simulink model "w3_warplab_trigger_proc"  (Simulink 7.7)
settings: Solver=ode45  StartTime=0.0  StopTime=100  RelTol=1e-3
InitFcn:
  | warplab_trigger_proc_init
StartFcn:
  | warplab_trigger_proc_init
undefined symbols (not defined in the file or in its folder): gcbh, xlBlockLoadCallback, xlGetNormalizedPeriod
libraries: xbsIndex_r4 x817, xbsEDKLib_r4 x1
(part 6 of 6)

== system w3_warplab_trigger_proc/Trigger Sources/Energy/AntD Detector/Idle Detection ==
  Avg RSSI : Inport
  Reset : Inport  Port=2
  en : Inport  Port=3
  Convert1 : xbsIndex_r4/Convert  gui_display_data_type=Fixed-point  arith_type=Unsigned  n_bits=1  bin_pt=0  float_type=Single  exp_bits=8  fraction_bits=24  quantization=Truncate  overflow=Wrap  en=off  latency=0  dbl_ovrd=off  pipeline=off  block_type=convert
      settings: block_version=VER_STRING_GOES_HERE
  Counter1 : xbsIndex_r4/Counter  cnt_type=Free Running  cnt_to=Inf  operation=Up  start_count=0  cnt_by_val=1  arith_type=Unsigned  n_bits=11  bin_pt=0  load_pin=off  rst=on  en=on  explicit_period=off  period=4  dbl_ovrd=off  use_behavioral_HDL=off  implementation=Fabric  use_rpm=off  block_type=counter
  Inverter1 : xbsIndex_r4/Inverter  en=off  latency=0  dbl_ovrd=off  block_type=inv
      settings: xl_area=[0 0 0 0 0 0 0]  block_version=8.2
  Logical : xbsIndex_r4/Logical  logical_function=AND  inputs=2  en=off  latency=0  precision=Full  arith_type=Unsigned  n_bits=16  bin_pt=0  align_bp=on  dbl_ovrd=off  block_type=logical
  Logical1 : xbsIndex_r4/Logical  logical_function=OR  inputs=2  en=off  latency=0  precision=Full  arith_type=Unsigned  n_bits=16  bin_pt=0  align_bp=on  dbl_ovrd=off  block_type=logical
  Relational2 : xbsIndex_r4/Relational  mode=a<b  en=off  latency=0  dbl_ovrd=off  block_type=relational
      settings: block_version=VER_STRING_GOES_HERE
  Relational3 : xbsIndex_r4/Relational  mode=a>b  en=off  latency=0  dbl_ovrd=off  block_type=relational
      settings: block_version=VER_STRING_GOES_HERE
  S-R Latch : Subsystem
  Idle : Outport
  wires:
  Convert1/1 -> Idle/1
  Avg RSSI/1 -> Relational2/1
  S-R Latch/1(Q) -> Convert1/1
  Relational3/1 -> S-R Latch/2(S)
  [pktDet_duration_idle] -> Relational3/2
  Counter1/1 -> Relational3/1
  Inverter1/1 -> Logical1/2
  Logical1/1 -> Counter1/1, S-R Latch/1(R)
  Reset/1 -> Logical1/1
  Relational2/1 -> Logical/1, Inverter1/1
  [pktDet_energyThresh_idle] -> Relational2/2
  en/1 -> Logical/2
  Logical/1 -> Counter1/2

== system w3_warplab_trigger_proc/Trigger Sources/Energy/AntD Detector/Running Sum ==
  note: This block impelemnts a variable-length running sum.
      | For a sum y(n) of the previous N samples of sequence x(n), it implements
      | y(n) = y(n-1) + x(n) - x(n-N)
      | This requires a careful reset procedure, where the full shift register
      | is zerored out. Otherwise the feedback-based sum stops working.
  RSSI : Inport
  reset : Inport  Port=2
  avglen : Inport  Port=3
  en : Inport  Port=4
  ASR : xbsIndex_r4/Addressable Shift Register  infer_latency=on  depth=2  initVector=[0]  en=on  dbl_ovrd=off  use_behavioral_HDL=off  Optimization=Resource  use_rpm=off  block_type=addrsr
      settings: infoedit="Delay of configurable length.  Any element in the delay line can be addressed and driven onto the output port.<br><br>Hardware notes: This block is implemented using SRL16s. If Virtex-4 or Spartan-3 device is used, multiple SRLC16s are cascaded together."  block_version=VER_STRING_GOES_HERE
  Accumulator : xbsIndex_r4/Accumulator  operation=Add  n_bits=17  overflow=Flag as error  scale=1  rst=on  infoeditControl=reset for floating point data type must be asserted for a minimum of 2 cycles  hasbypass=off  en=on  latency=0  dbl_ovrd=off  msb_inp=100  msb=100  lsb=-100  use_behavioral_HDL=on  implementation=Fabric  block_type=accum
      settings: block_version=VER_STRING_GOES_HERE
  AddSub : xbsIndex_r4/AddSub  mode=Subtraction  use_carryin=off  use_carryout=off  en=off  latency=0  precision=Full  arith_type=Unsigned  n_bits=10  bin_pt=0  quantization=Truncate  overflow=Wrap  dbl_ovrd=off  use_behavioral_HDL=off  hw_selection=Fabric  pipelined=off  use_rpm=on  block_type=addsub
      settings: block_version=VER_STRING_GOES_HERE
  Convert7 : xbsIndex_r4/Convert  gui_display_data_type=Fixed-point  arith_type=Unsigned  n_bits=17  bin_pt=0  float_type=Single  exp_bits=8  fraction_bits=24  quantization=Truncate  overflow=Saturate  en=off  latency=0  dbl_ovrd=off  pipeline=off  block_type=convert
      settings: block_version=10.1.3
  Logical : xbsIndex_r4/Logical  logical_function=OR  inputs=2  en=off  latency=0  precision=Full  arith_type=Unsigned  n_bits=16  bin_pt=0  align_bp=on  dbl_ovrd=off  block_type=logical
  Long Reset Gen : Subsystem
  Register : xbsIndex_r4/Register  init=0  rst=on  en=off  dbl_ovrd=off  block_type=register
      settings: block_version=VER_STRING_GOES_HERE
  avg : Outport
  wires:
  en/1 -> Accumulator/3, ASR/3
  Convert7/1 -> avg/1
  Long Reset Gen/1(reset_out) -> Logical/1
  reset/1 -> Logical/2, Long Reset Gen/2(reset_in)
  Logical/1 -> Accumulator/2, Register/2
  Accumulator/1 -> Convert7/1
  RSSI/1 -> Register/1
  avglen/1 -> Long Reset Gen/1(duration), ASR/2
  Register/1 -> AddSub/1, ASR/1
  AddSub/1 -> Accumulator/1
  ASR/1 -> AddSub/2

== system w3_warplab_trigger_proc/Trigger Sources/Ethernet/Pkt Comp/Output Reg 0 ==
  Match : Inport
  Done : Inport  Port=2
  Delay2 : xbsIndex_r4/Delay  rst=off  infoeditControl=Selection of Reset will increase slice count due to use of real FFs and instead of SRLs  en=off  latency=32  dbl_ovrd=off  reg_retiming=off  block_type=delay
  Register : xbsIndex_r4/Register  init=0  rst=on  en=on  dbl_ovrd=off  block_type=register
  Out : Outport
  wires:
  Delay2/1 -> Register/2
  Register/1 -> Out/1
  Match/1 -> Register/1
  Done/1 -> Delay2/1, Register/3

== system w3_warplab_trigger_proc/Trigger Sources/Ethernet/Pkt Comp/Pkt Match ==
  Valid : Inport
  Word Match : Inport  Port=2
  Reset : Inport  Port=3
  Inverter1 : xbsIndex_r4/Inverter  en=off  latency=0  dbl_ovrd=off  block_type=inv
  Inverter2 : xbsIndex_r4/Inverter  en=off  latency=0  dbl_ovrd=off  block_type=inv
  Logical3 : xbsIndex_r4/Logical  logical_function=AND  inputs=2  en=off  latency=0  precision=Full  arith_type=Unsigned  n_bits=16  bin_pt=0  align_bp=on  dbl_ovrd=off  block_type=logical
  Pkt Match Fail : Subsystem
  Pkt Match : Outport
  wires:
  Logical3/1 -> Pkt Match Fail/1(S)
  Inverter1/1 -> Logical3/2
  Pkt Match Fail/1(Q) -> Inverter2/1
  Valid/1 -> Logical3/1
  Word Match/1 -> Inverter1/1
  Inverter2/1 -> Pkt Match/1
  Reset/1 -> Pkt Match Fail/2(R)

== system w3_warplab_trigger_proc/Trigger Sources/Ethernet/Pkt Comp/Word Comp 0 ==
  note: No state in this block- Each word is compared
      | with zero latency. All per-packet state must
      | be maintained elsewhere.
  Word Addr : Inport
  TDATA : Inport  Port=2
  Byte Comp 0 : Subsystem
  Byte Comp 1 : Subsystem
  Byte Comp 2 : Subsystem
  Byte Comp 3 : Subsystem
  Constant1 : xbsIndex_r4/Constant  const=0  gui_display_data_type=Fixed-point  arith_type=Unsigned  n_bits=32  bin_pt=0  preci_type=Single  exp_width=8  frac_width=24  explicit_period=off  period=1  equ=P=C  opselect=C  inp2=PCIN>>17  opr=+  inp1=P  carry=CIN  dbl_ovrd=off  block_type=constant
  Constant2 : xbsIndex_r4/Constant  const=0  gui_display_data_type=Fixed-point  arith_type=Unsigned  n_bits=32  bin_pt=0  preci_type=Single  exp_width=8  frac_width=24  explicit_period=off  period=1  equ=P=C  opselect=C  inp2=PCIN>>17  opr=+  inp1=P  carry=CIN  dbl_ovrd=off  block_type=constant
  Constant3 : xbsIndex_r4/Constant  const=0  gui_display_data_type=Boolean  arith_type=Boolean  n_bits=1  bin_pt=0  preci_type=Single  exp_width=8  frac_width=24  explicit_period=off  period=1  equ=P=C  opselect=C  inp2=PCIN>>17  opr=+  inp1=P  carry=CIN  dbl_ovrd=off  block_type=constant
  Constant5 : xbsIndex_r4/Constant  const=0  gui_display_data_type=Boolean  arith_type=Boolean  n_bits=1  bin_pt=0  preci_type=Single  exp_width=8  frac_width=24  explicit_period=off  period=1  equ=P=C  opselect=C  inp2=PCIN>>17  opr=+  inp1=P  carry=CIN  dbl_ovrd=off  block_type=constant
  Logical : xbsIndex_r4/Logical  logical_function=AND  inputs=4  en=off  latency=0  precision=Full  arith_type=Unsigned  n_bits=16  bin_pt=0  align_bp=on  dbl_ovrd=off  block_type=logical
  Logical1 : xbsIndex_r4/Logical  logical_function=OR  inputs=4  en=off  latency=0  precision=Full  arith_type=Unsigned  n_bits=16  bin_pt=0  align_bp=on  dbl_ovrd=off  block_type=logical
  Logical2 : xbsIndex_r4/Logical  logical_function=AND  inputs=4  en=off  latency=0  precision=Full  arith_type=Unsigned  n_bits=16  bin_pt=0  align_bp=on  dbl_ovrd=off  block_type=logical
  Mux1 : xbsIndex_r4/Mux  inputs=2  en=off  latency=0  precision=Full  arith_type=Unsigned  n_bits=16  bin_pt=14  quantization=Truncate  overflow=Wrap  dbl_ovrd=off  block_type=mux
  Shared Memory1 : xbsIndex_r4/Shared Memory  shared_memory_name='PktTemplate0'  depth=64  ownership=Locally Owned and Initialized  initVector=0  en=off  mutex=Unprotected  mode=Read and Write  write_mode=Read After Write  time_out=0  latency=1  explicit_data_type=on  gui_display_data_type=Fixed-point  arith_type=Unsigned  n_bits=32  bin_pt=0  preci_type=Single  implementation=Block RAM  use_rpm=off  block_type=shmem
      settings: AttributesFormatString=<< %<shared_memory_name> >>
  Shared Memory2 : xbsIndex_r4/Shared Memory  shared_memory_name='PktOps0'  depth=64  ownership=Locally Owned and Initialized  initVector=0  en=off  mutex=Unprotected  mode=Read and Write  write_mode=Read After Write  time_out=0  latency=1  explicit_data_type=on  gui_display_data_type=Fixed-point  arith_type=Unsigned  n_bits=32  bin_pt=0  preci_type=Single  implementation=Block RAM  use_rpm=off  block_type=shmem
      settings: AttributesFormatString=<< %<shared_memory_name> >>
  Subsystem : Subsystem
  Subsystem1 : Subsystem
  Subsystem2 : Subsystem
  Word Match : Outport
  wires:
  Constant3/1 -> Shared Memory1/3
  Constant2/1 -> Shared Memory1/2
  Word Addr/1 -> Shared Memory1/1, Shared Memory2/1
  Constant1/1 -> Shared Memory2/2
  Constant5/1 -> Shared Memory2/3
  Shared Memory2/1 -> Subsystem/1(32b)
  Shared Memory1/1 -> Subsystem1/1(32b)
  TDATA/1 -> Subsystem2/1(32b)
  Subsystem2/1(B0) -> Byte Comp 0/1(Data)
  Subsystem/1(B0) -> Byte Comp 0/2(Op)
  Subsystem1/1(B0) -> Byte Comp 0/3(Template)
  Subsystem2/2(B1) -> Byte Comp 1/1(Data)
  Subsystem/2(B1) -> Byte Comp 1/2(Op)
  Subsystem1/2(B1) -> Byte Comp 1/3(Template)
  Subsystem1/3(B2) -> Byte Comp 2/3(Template)
  Subsystem/3(B2) -> Byte Comp 2/2(Op)
  Subsystem2/3(B2) -> Byte Comp 2/1(Data)
  Subsystem2/4(B3) -> Byte Comp 3/1(Data)
  Subsystem/4(B3) -> Byte Comp 3/2(Op)
  Subsystem1/4(B3) -> Byte Comp 3/3(Template)
  Logical/1 -> Mux1/2
  Logical1/1 -> Mux1/3
  Logical2/1 -> Mux1/1
  Byte Comp 2/2(Or Op) -> Logical2/3
  Byte Comp 3/2(Or Op) -> Logical2/4
  Byte Comp 0/2(Or Op) -> Logical2/1
  Byte Comp 1/2(Or Op) -> Logical2/2
  Byte Comp 0/1(Res) -> Logical/1, Logical1/1
  Byte Comp 1/1(Res) -> Logical1/2, Logical/2
  Byte Comp 2/1(Res) -> Logical/3, Logical1/3
  Byte Comp 3/1(Res) -> Logical/4, Logical1/4
  Mux1/1 -> Word Match/1

== system w3_warplab_trigger_proc/Trigger Sources/Energy/AntA Detector/Busy Detection/S-R Latch ==
  R : Inport
  S : Inport  Port=2
  Constant1 : xbsIndex_r4/Constant  const=1  gui_display_data_type=Fixed-point  arith_type=Boolean  n_bits=1  bin_pt=0  preci_type=Single  exp_width=8  frac_width=24  explicit_period=off  period=1  equ=P=C  opselect=C  inp2=PCIN>>17  opr=+  inp1=P  carry=CIN  dbl_ovrd=off  block_type=constant
      settings: block_version=VER_STRING_GOES_HERE
  Register2 : xbsIndex_r4/Register  init=0  rst=on  en=on  dbl_ovrd=off  block_type=register
      settings: xl_area=[1 1 0 0 0 0 0]  block_version=VER_STRING_GOES_HERE
  Q : Outport
  wires:
  Constant1/1 -> Register2/1
  R/1 -> Register2/2
  Register2/1 -> Q/1
  S/1 -> Register2/3

== system w3_warplab_trigger_proc/Trigger Sources/Energy/AntA Detector/Idle Detection/S-R Latch ==
  R : Inport
  S : Inport  Port=2
  Constant1 : xbsIndex_r4/Constant  const=1  gui_display_data_type=Fixed-point  arith_type=Boolean  n_bits=1  bin_pt=0  preci_type=Single  exp_width=8  frac_width=24  explicit_period=off  period=1  equ=P=C  opselect=C  inp2=PCIN>>17  opr=+  inp1=P  carry=CIN  dbl_ovrd=off  block_type=constant
      settings: block_version=VER_STRING_GOES_HERE
  Register2 : xbsIndex_r4/Register  init=0  rst=on  en=on  dbl_ovrd=off  block_type=register
      settings: xl_area=[1 1 0 0 0 0 0]  block_version=VER_STRING_GOES_HERE
  Q : Outport
  wires:
  S/1 -> Register2/3
  Register2/1 -> Q/1
  R/1 -> Register2/2
  Constant1/1 -> Register2/1

== system w3_warplab_trigger_proc/Trigger Sources/Energy/AntA Detector/Running Sum/Long Reset Gen ==
  duration : Inport
  reset_in : Inport  Port=2
  Counter : xbsIndex_r4/Counter  cnt_type=Free Running  cnt_to=0  operation=Up  start_count=0  cnt_by_val=1  arith_type=Unsigned  n_bits=8  bin_pt=0  load_pin=off  rst=on  en=on  explicit_period=off  period=4  dbl_ovrd=off  use_behavioral_HDL=off  implementation=Fabric  use_rpm=off  block_type=counter
      settings: block_version=VER_STRING_GOES_HERE
  Relational : xbsIndex_r4/Relational  mode=a=b  en=off  latency=0  dbl_ovrd=off  block_type=relational
      settings: block_version=VER_STRING_GOES_HERE
  S-R Latch : Subsystem
  reset_out : Outport
  wires:
  Relational/1 -> Counter/1, S-R Latch/2(R)
  Counter/1 -> Relational/1
  reset_in/1 -> S-R Latch/1(S)
  duration/1 -> Relational/2
  S-R Latch/1(Q) -> Counter/2, reset_out/1

== system w3_warplab_trigger_proc/Trigger Sources/Energy/AntB Detector/Busy Detection/S-R Latch ==
  R : Inport
  S : Inport  Port=2
  Constant1 : xbsIndex_r4/Constant  const=1  gui_display_data_type=Fixed-point  arith_type=Boolean  n_bits=1  bin_pt=0  preci_type=Single  exp_width=8  frac_width=24  explicit_period=off  period=1  equ=P=C  opselect=C  inp2=PCIN>>17  opr=+  inp1=P  carry=CIN  dbl_ovrd=off  block_type=constant
      settings: block_version=VER_STRING_GOES_HERE
  Register2 : xbsIndex_r4/Register  init=0  rst=on  en=on  dbl_ovrd=off  block_type=register
      settings: xl_area=[1 1 0 0 0 0 0]  block_version=VER_STRING_GOES_HERE
  Q : Outport
  wires:
  Constant1/1 -> Register2/1
  R/1 -> Register2/2
  Register2/1 -> Q/1
  S/1 -> Register2/3

== system w3_warplab_trigger_proc/Trigger Sources/Energy/AntB Detector/Idle Detection/S-R Latch ==
  R : Inport
  S : Inport  Port=2
  Constant1 : xbsIndex_r4/Constant  const=1  gui_display_data_type=Fixed-point  arith_type=Boolean  n_bits=1  bin_pt=0  preci_type=Single  exp_width=8  frac_width=24  explicit_period=off  period=1  equ=P=C  opselect=C  inp2=PCIN>>17  opr=+  inp1=P  carry=CIN  dbl_ovrd=off  block_type=constant
      settings: block_version=VER_STRING_GOES_HERE
  Register2 : xbsIndex_r4/Register  init=0  rst=on  en=on  dbl_ovrd=off  block_type=register
      settings: xl_area=[1 1 0 0 0 0 0]  block_version=VER_STRING_GOES_HERE
  Q : Outport
  wires:
  S/1 -> Register2/3
  Register2/1 -> Q/1
  R/1 -> Register2/2
  Constant1/1 -> Register2/1

== system w3_warplab_trigger_proc/Trigger Sources/Energy/AntB Detector/Running Sum/Long Reset Gen ==
  duration : Inport
  reset_in : Inport  Port=2
  Counter : xbsIndex_r4/Counter  cnt_type=Free Running  cnt_to=0  operation=Up  start_count=0  cnt_by_val=1  arith_type=Unsigned  n_bits=8  bin_pt=0  load_pin=off  rst=on  en=on  explicit_period=off  period=4  dbl_ovrd=off  use_behavioral_HDL=off  implementation=Fabric  use_rpm=off  block_type=counter
      settings: block_version=VER_STRING_GOES_HERE
  Relational : xbsIndex_r4/Relational  mode=a=b  en=off  latency=0  dbl_ovrd=off  block_type=relational
      settings: block_version=VER_STRING_GOES_HERE
  S-R Latch : Subsystem
  reset_out : Outport
  wires:
  S-R Latch/1(Q) -> reset_out/1, Counter/2
  duration/1 -> Relational/2
  reset_in/1 -> S-R Latch/1(S)
  Counter/1 -> Relational/1
  Relational/1 -> S-R Latch/2(R), Counter/1

== system w3_warplab_trigger_proc/Trigger Sources/Energy/AntC Detector/Busy Detection/S-R Latch ==
  R : Inport
  S : Inport  Port=2
  Constant1 : xbsIndex_r4/Constant  const=1  gui_display_data_type=Fixed-point  arith_type=Boolean  n_bits=1  bin_pt=0  preci_type=Single  exp_width=8  frac_width=24  explicit_period=off  period=1  equ=P=C  opselect=C  inp2=PCIN>>17  opr=+  inp1=P  carry=CIN  dbl_ovrd=off  block_type=constant
      settings: block_version=VER_STRING_GOES_HERE
  Register2 : xbsIndex_r4/Register  init=0  rst=on  en=on  dbl_ovrd=off  block_type=register
      settings: xl_area=[1 1 0 0 0 0 0]  block_version=VER_STRING_GOES_HERE
  Q : Outport
  wires:
  Constant1/1 -> Register2/1
  R/1 -> Register2/2
  Register2/1 -> Q/1
  S/1 -> Register2/3

== system w3_warplab_trigger_proc/Trigger Sources/Energy/AntC Detector/Idle Detection/S-R Latch ==
  R : Inport
  S : Inport  Port=2
  Constant1 : xbsIndex_r4/Constant  const=1  gui_display_data_type=Fixed-point  arith_type=Boolean  n_bits=1  bin_pt=0  preci_type=Single  exp_width=8  frac_width=24  explicit_period=off  period=1  equ=P=C  opselect=C  inp2=PCIN>>17  opr=+  inp1=P  carry=CIN  dbl_ovrd=off  block_type=constant
      settings: block_version=VER_STRING_GOES_HERE
  Register2 : xbsIndex_r4/Register  init=0  rst=on  en=on  dbl_ovrd=off  block_type=register
      settings: xl_area=[1 1 0 0 0 0 0]  block_version=VER_STRING_GOES_HERE
  Q : Outport
  wires:
  S/1 -> Register2/3
  Register2/1 -> Q/1
  R/1 -> Register2/2
  Constant1/1 -> Register2/1

== system w3_warplab_trigger_proc/Trigger Sources/Energy/AntC Detector/Running Sum/Long Reset Gen ==
  duration : Inport
  reset_in : Inport  Port=2
  Counter : xbsIndex_r4/Counter  cnt_type=Free Running  cnt_to=0  operation=Up  start_count=0  cnt_by_val=1  arith_type=Unsigned  n_bits=8  bin_pt=0  load_pin=off  rst=on  en=on  explicit_period=off  period=4  dbl_ovrd=off  use_behavioral_HDL=off  implementation=Fabric  use_rpm=off  block_type=counter
      settings: block_version=VER_STRING_GOES_HERE
  Relational : xbsIndex_r4/Relational  mode=a=b  en=off  latency=0  dbl_ovrd=off  block_type=relational
      settings: block_version=VER_STRING_GOES_HERE
  S-R Latch : Subsystem
  reset_out : Outport
  wires:
  Relational/1 -> Counter/1, S-R Latch/2(R)
  Counter/1 -> Relational/1
  reset_in/1 -> S-R Latch/1(S)
  duration/1 -> Relational/2
  S-R Latch/1(Q) -> Counter/2, reset_out/1

== system w3_warplab_trigger_proc/Trigger Sources/Energy/AntD Detector/Busy Detection/S-R Latch ==
  R : Inport
  S : Inport  Port=2
  Constant1 : xbsIndex_r4/Constant  const=1  gui_display_data_type=Fixed-point  arith_type=Boolean  n_bits=1  bin_pt=0  preci_type=Single  exp_width=8  frac_width=24  explicit_period=off  period=1  equ=P=C  opselect=C  inp2=PCIN>>17  opr=+  inp1=P  carry=CIN  dbl_ovrd=off  block_type=constant
      settings: block_version=VER_STRING_GOES_HERE
  Register2 : xbsIndex_r4/Register  init=0  rst=on  en=on  dbl_ovrd=off  block_type=register
      settings: xl_area=[1 1 0 0 0 0 0]  block_version=VER_STRING_GOES_HERE
  Q : Outport
  wires:
  Constant1/1 -> Register2/1
  R/1 -> Register2/2
  Register2/1 -> Q/1
  S/1 -> Register2/3

== system w3_warplab_trigger_proc/Trigger Sources/Energy/AntD Detector/Idle Detection/S-R Latch ==
  R : Inport
  S : Inport  Port=2
  Constant1 : xbsIndex_r4/Constant  const=1  gui_display_data_type=Fixed-point  arith_type=Boolean  n_bits=1  bin_pt=0  preci_type=Single  exp_width=8  frac_width=24  explicit_period=off  period=1  equ=P=C  opselect=C  inp2=PCIN>>17  opr=+  inp1=P  carry=CIN  dbl_ovrd=off  block_type=constant
      settings: block_version=VER_STRING_GOES_HERE
  Register2 : xbsIndex_r4/Register  init=0  rst=on  en=on  dbl_ovrd=off  block_type=register
      settings: xl_area=[1 1 0 0 0 0 0]  block_version=VER_STRING_GOES_HERE
  Q : Outport
  wires:
  S/1 -> Register2/3
  Register2/1 -> Q/1
  R/1 -> Register2/2
  Constant1/1 -> Register2/1

== system w3_warplab_trigger_proc/Trigger Sources/Energy/AntD Detector/Running Sum/Long Reset Gen ==
  duration : Inport
  reset_in : Inport  Port=2
  Counter : xbsIndex_r4/Counter  cnt_type=Free Running  cnt_to=0  operation=Up  start_count=0  cnt_by_val=1  arith_type=Unsigned  n_bits=8  bin_pt=0  load_pin=off  rst=on  en=on  explicit_period=off  period=4  dbl_ovrd=off  use_behavioral_HDL=off  implementation=Fabric  use_rpm=off  block_type=counter
      settings: block_version=VER_STRING_GOES_HERE
  Relational : xbsIndex_r4/Relational  mode=a=b  en=off  latency=0  dbl_ovrd=off  block_type=relational
      settings: block_version=VER_STRING_GOES_HERE
  S-R Latch : Subsystem
  reset_out : Outport
  wires:
  S-R Latch/1(Q) -> reset_out/1, Counter/2
  duration/1 -> Relational/2
  reset_in/1 -> S-R Latch/1(S)
  Counter/1 -> Relational/1
  Relational/1 -> S-R Latch/2(R), Counter/1

== system w3_warplab_trigger_proc/Trigger Sources/Ethernet/Pkt Comp/Pkt Match/Pkt Match Fail ==
  S : Inport
  R : Inport  Port=2
  Constant5 : xbsIndex_r4/Constant  const=1  gui_display_data_type=Fixed-point  arith_type=Unsigned  n_bits=1  bin_pt=0  preci_type=Single  exp_width=8  frac_width=24  explicit_period=off  period=1  equ=P=C  opselect=C  inp2=PCIN>>17  opr=+  inp1=P  carry=CIN  dbl_ovrd=off  block_type=constant
  Convert : xbsIndex_r4/Convert  gui_display_data_type=Boolean  arith_type=Boolean  n_bits=16  bin_pt=14  float_type=Single  exp_bits=8  fraction_bits=24  quantization=Truncate  overflow=Wrap  en=off  latency=0  dbl_ovrd=off  pipeline=off  block_type=convert
  Convert1 : xbsIndex_r4/Convert  gui_display_data_type=Boolean  arith_type=Boolean  n_bits=16  bin_pt=14  float_type=Single  exp_bits=8  fraction_bits=24  quantization=Truncate  overflow=Wrap  en=off  latency=0  dbl_ovrd=off  pipeline=off  block_type=convert
  Register : xbsIndex_r4/Register  init=0  rst=on  en=on  dbl_ovrd=off  block_type=register
  Q : Outport
  wires:
  Constant5/1 -> Register/1
  R/1 -> Convert/1
  Register/1 -> Q/1
  S/1 -> Convert1/1
  Convert/1 -> Register/2
  Convert1/1 -> Register/3

== system w3_warplab_trigger_proc/Trigger Sources/Ethernet/Pkt Comp/Word Comp 0/Byte Comp 0 ==
  note: Valid Op Codes:
      | 0: Don't care (always match)
      | 1: Equal (all bits match)
      | 2: Not-equal (>0 bits don't match)
      | 3: Any bit matches (AND(T,D)>0)
  Data : Inport
  Op : Inport  Port=2
  Template : Inport  Port=3
  2LSB : xbsIndex_r4/Slice  nbits=2  boolean_output=off  mode=Lower Bit Location + Width  bit1=0  base1=MSB of Input  bit0=0  base0=LSB of Input  dbl_ovrd=off  block_type=slice
  Any of AND : Subsystem
  Constant : xbsIndex_r4/Constant  const=1  gui_display_data_type=Boolean  arith_type=Boolean  n_bits=16  bin_pt=14  preci_type=Single  exp_width=8  frac_width=24  explicit_period=off  period=1  equ=P=C  opselect=C  inp2=PCIN>>17  opr=+  inp1=P  carry=CIN  dbl_ovrd=off  block_type=constant
  Constant1 : xbsIndex_r4/Constant  const=0  gui_display_data_type=Fixed-point  arith_type=Unsigned  n_bits=1  bin_pt=0  preci_type=Single  exp_width=8  frac_width=24  explicit_period=off  period=1  equ=P=C  opselect=C  inp2=PCIN>>17  opr=+  inp1=P  carry=CIN  dbl_ovrd=off  block_type=constant
  Constant2 : xbsIndex_r4/Constant  const=0  gui_display_data_type=Fixed-point  arith_type=Unsigned  n_bits=1  bin_pt=0  preci_type=Single  exp_width=8  frac_width=24  explicit_period=off  period=1  equ=P=C  opselect=C  inp2=PCIN>>17  opr=+  inp1=P  carry=CIN  dbl_ovrd=off  block_type=constant
  Constant3 : xbsIndex_r4/Constant  const=0  gui_display_data_type=Fixed-point  arith_type=Unsigned  n_bits=1  bin_pt=0  preci_type=Single  exp_width=8  frac_width=24  explicit_period=off  period=1  equ=P=C  opselect=C  inp2=PCIN>>17  opr=+  inp1=P  carry=CIN  dbl_ovrd=off  block_type=constant
  Constant4 : xbsIndex_r4/Constant  const=1  gui_display_data_type=Fixed-point  arith_type=Unsigned  n_bits=1  bin_pt=0  preci_type=Single  exp_width=8  frac_width=24  explicit_period=off  period=1  equ=P=C  opselect=C  inp2=PCIN>>17  opr=+  inp1=P  carry=CIN  dbl_ovrd=off  block_type=constant
  Equal : Subsystem
  Mux : xbsIndex_r4/Mux  inputs=4  en=off  latency=0  precision=Full  arith_type=Unsigned  n_bits=16  bin_pt=14  quantization=Truncate  overflow=Wrap  dbl_ovrd=off  block_type=mux
  Mux1 : xbsIndex_r4/Mux  inputs=4  en=off  latency=0  precision=Full  arith_type=Unsigned  n_bits=16  bin_pt=14  quantization=Truncate  overflow=Wrap  dbl_ovrd=off  block_type=mux
  Not Equal : Subsystem
  Res : Outport
  Or Op : Outport  Port=2
  wires:
  Op/1 -> 2LSB/1
  Mux/1 -> Res/1
  Constant/1 -> Mux/2
  Equal/1(R) -> Mux/3
  Not Equal/1(R) -> Mux/4
  Any of AND/1(R) -> Mux/5
  Data/1 -> Equal/1(D), Not Equal/1(D), Any of AND/1(D)
  Template/1 -> Equal/2(BT), Not Equal/2(BT), Any of AND/2(T)
  2LSB/1 -> Mux/1, Mux1/1
  Mux1/1 -> Or Op/1
  Constant1/1 -> Mux1/2
  Constant2/1 -> Mux1/3
  Constant3/1 -> Mux1/4
  Constant4/1 -> Mux1/5

== system w3_warplab_trigger_proc/Trigger Sources/Ethernet/Pkt Comp/Word Comp 0/Byte Comp 1 ==
  note: Valid Op Codes:
      | 0: Don't care (always match)
      | 1: Equal (all bits match)
      | 2: Not-equal (>0 bits don't match)
      | 3: Any bit matches (AND(T,D)>0)
  Data : Inport
  Op : Inport  Port=2
  Template : Inport  Port=3
  2LSB : xbsIndex_r4/Slice  nbits=2  boolean_output=off  mode=Lower Bit Location + Width  bit1=0  base1=MSB of Input  bit0=0  base0=LSB of Input  dbl_ovrd=off  block_type=slice
  Any of AND : Subsystem
  Constant : xbsIndex_r4/Constant  const=1  gui_display_data_type=Boolean  arith_type=Boolean  n_bits=16  bin_pt=14  preci_type=Single  exp_width=8  frac_width=24  explicit_period=off  period=1  equ=P=C  opselect=C  inp2=PCIN>>17  opr=+  inp1=P  carry=CIN  dbl_ovrd=off  block_type=constant
  Constant1 : xbsIndex_r4/Constant  const=0  gui_display_data_type=Fixed-point  arith_type=Unsigned  n_bits=1  bin_pt=0  preci_type=Single  exp_width=8  frac_width=24  explicit_period=off  period=1  equ=P=C  opselect=C  inp2=PCIN>>17  opr=+  inp1=P  carry=CIN  dbl_ovrd=off  block_type=constant
  Constant2 : xbsIndex_r4/Constant  const=0  gui_display_data_type=Fixed-point  arith_type=Unsigned  n_bits=1  bin_pt=0  preci_type=Single  exp_width=8  frac_width=24  explicit_period=off  period=1  equ=P=C  opselect=C  inp2=PCIN>>17  opr=+  inp1=P  carry=CIN  dbl_ovrd=off  block_type=constant
  Constant3 : xbsIndex_r4/Constant  const=0  gui_display_data_type=Fixed-point  arith_type=Unsigned  n_bits=1  bin_pt=0  preci_type=Single  exp_width=8  frac_width=24  explicit_period=off  period=1  equ=P=C  opselect=C  inp2=PCIN>>17  opr=+  inp1=P  carry=CIN  dbl_ovrd=off  block_type=constant
  Constant4 : xbsIndex_r4/Constant  const=1  gui_display_data_type=Fixed-point  arith_type=Unsigned  n_bits=1  bin_pt=0  preci_type=Single  exp_width=8  frac_width=24  explicit_period=off  period=1  equ=P=C  opselect=C  inp2=PCIN>>17  opr=+  inp1=P  carry=CIN  dbl_ovrd=off  block_type=constant
  Equal : Subsystem
  Mux : xbsIndex_r4/Mux  inputs=4  en=off  latency=0  precision=Full  arith_type=Unsigned  n_bits=16  bin_pt=14  quantization=Truncate  overflow=Wrap  dbl_ovrd=off  block_type=mux
  Mux1 : xbsIndex_r4/Mux  inputs=4  en=off  latency=0  precision=Full  arith_type=Unsigned  n_bits=16  bin_pt=14  quantization=Truncate  overflow=Wrap  dbl_ovrd=off  block_type=mux
  Not Equal : Subsystem
  Res : Outport
  Or Op : Outport  Port=2
  wires:
  Constant4/1 -> Mux1/5
  Constant3/1 -> Mux1/4
  Constant2/1 -> Mux1/3
  Constant1/1 -> Mux1/2
  Mux1/1 -> Or Op/1
  2LSB/1 -> Mux1/1, Mux/1
  Template/1 -> Any of AND/2(T), Not Equal/2(BT), Equal/2(BT)
  Data/1 -> Any of AND/1(D), Not Equal/1(D), Equal/1(D)
  Any of AND/1(R) -> Mux/5
  Not Equal/1(R) -> Mux/4
  Equal/1(R) -> Mux/3
  Constant/1 -> Mux/2
  Mux/1 -> Res/1
  Op/1 -> 2LSB/1

== system w3_warplab_trigger_proc/Trigger Sources/Ethernet/Pkt Comp/Word Comp 0/Byte Comp 2 ==
  note: Valid Op Codes:
      | 0: Don't care (always match)
      | 1: Equal (all bits match)
      | 2: Not-equal (>0 bits don't match)
      | 3: Any bit matches (AND(T,D)>0)
  Data : Inport
  Op : Inport  Port=2
  Template : Inport  Port=3
  2LSB : xbsIndex_r4/Slice  nbits=2  boolean_output=off  mode=Lower Bit Location + Width  bit1=0  base1=MSB of Input  bit0=0  base0=LSB of Input  dbl_ovrd=off  block_type=slice
  Any of AND : Subsystem
  Constant : xbsIndex_r4/Constant  const=1  gui_display_data_type=Boolean  arith_type=Boolean  n_bits=16  bin_pt=14  preci_type=Single  exp_width=8  frac_width=24  explicit_period=off  period=1  equ=P=C  opselect=C  inp2=PCIN>>17  opr=+  inp1=P  carry=CIN  dbl_ovrd=off  block_type=constant
  Constant1 : xbsIndex_r4/Constant  const=0  gui_display_data_type=Fixed-point  arith_type=Unsigned  n_bits=1  bin_pt=0  preci_type=Single  exp_width=8  frac_width=24  explicit_period=off  period=1  equ=P=C  opselect=C  inp2=PCIN>>17  opr=+  inp1=P  carry=CIN  dbl_ovrd=off  block_type=constant
  Constant2 : xbsIndex_r4/Constant  const=0  gui_display_data_type=Fixed-point  arith_type=Unsigned  n_bits=1  bin_pt=0  preci_type=Single  exp_width=8  frac_width=24  explicit_period=off  period=1  equ=P=C  opselect=C  inp2=PCIN>>17  opr=+  inp1=P  carry=CIN  dbl_ovrd=off  block_type=constant
  Constant3 : xbsIndex_r4/Constant  const=0  gui_display_data_type=Fixed-point  arith_type=Unsigned  n_bits=1  bin_pt=0  preci_type=Single  exp_width=8  frac_width=24  explicit_period=off  period=1  equ=P=C  opselect=C  inp2=PCIN>>17  opr=+  inp1=P  carry=CIN  dbl_ovrd=off  block_type=constant
  Constant4 : xbsIndex_r4/Constant  const=1  gui_display_data_type=Fixed-point  arith_type=Unsigned  n_bits=1  bin_pt=0  preci_type=Single  exp_width=8  frac_width=24  explicit_period=off  period=1  equ=P=C  opselect=C  inp2=PCIN>>17  opr=+  inp1=P  carry=CIN  dbl_ovrd=off  block_type=constant
  Equal : Subsystem
  Mux : xbsIndex_r4/Mux  inputs=4  en=off  latency=0  precision=Full  arith_type=Unsigned  n_bits=16  bin_pt=14  quantization=Truncate  overflow=Wrap  dbl_ovrd=off  block_type=mux
  Mux1 : xbsIndex_r4/Mux  inputs=4  en=off  latency=0  precision=Full  arith_type=Unsigned  n_bits=16  bin_pt=14  quantization=Truncate  overflow=Wrap  dbl_ovrd=off  block_type=mux
  Not Equal : Subsystem
  Res : Outport
  Or Op : Outport  Port=2
  wires:
  Op/1 -> 2LSB/1
  Mux/1 -> Res/1
  Constant/1 -> Mux/2
  Equal/1(R) -> Mux/3
  Not Equal/1(R) -> Mux/4
  Any of AND/1(R) -> Mux/5
  Data/1 -> Equal/1(D), Not Equal/1(D), Any of AND/1(D)
  Template/1 -> Equal/2(BT), Not Equal/2(BT), Any of AND/2(T)
  2LSB/1 -> Mux/1, Mux1/1
  Mux1/1 -> Or Op/1
  Constant1/1 -> Mux1/2
  Constant2/1 -> Mux1/3
  Constant3/1 -> Mux1/4
  Constant4/1 -> Mux1/5

== system w3_warplab_trigger_proc/Trigger Sources/Ethernet/Pkt Comp/Word Comp 0/Byte Comp 3 ==
  note: Valid Op Codes:
      | 0: Don't care (always match)
      | 1: Equal (all bits match)
      | 2: Not-equal (>0 bits don't match)
      | 3: Any bit matches (AND(T,D)>0)
  Data : Inport
  Op : Inport  Port=2
  Template : Inport  Port=3
  2LSB : xbsIndex_r4/Slice  nbits=2  boolean_output=off  mode=Lower Bit Location + Width  bit1=0  base1=MSB of Input  bit0=0  base0=LSB of Input  dbl_ovrd=off  block_type=slice
  Any of AND : Subsystem
  Constant : xbsIndex_r4/Constant  const=1  gui_display_data_type=Boolean  arith_type=Boolean  n_bits=16  bin_pt=14  preci_type=Single  exp_width=8  frac_width=24  explicit_period=off  period=1  equ=P=C  opselect=C  inp2=PCIN>>17  opr=+  inp1=P  carry=CIN  dbl_ovrd=off  block_type=constant
  Constant1 : xbsIndex_r4/Constant  const=0  gui_display_data_type=Fixed-point  arith_type=Unsigned  n_bits=1  bin_pt=0  preci_type=Single  exp_width=8  frac_width=24  explicit_period=off  period=1  equ=P=C  opselect=C  inp2=PCIN>>17  opr=+  inp1=P  carry=CIN  dbl_ovrd=off  block_type=constant
  Constant2 : xbsIndex_r4/Constant  const=0  gui_display_data_type=Fixed-point  arith_type=Unsigned  n_bits=1  bin_pt=0  preci_type=Single  exp_width=8  frac_width=24  explicit_period=off  period=1  equ=P=C  opselect=C  inp2=PCIN>>17  opr=+  inp1=P  carry=CIN  dbl_ovrd=off  block_type=constant
  Constant3 : xbsIndex_r4/Constant  const=0  gui_display_data_type=Fixed-point  arith_type=Unsigned  n_bits=1  bin_pt=0  preci_type=Single  exp_width=8  frac_width=24  explicit_period=off  period=1  equ=P=C  opselect=C  inp2=PCIN>>17  opr=+  inp1=P  carry=CIN  dbl_ovrd=off  block_type=constant
  Constant4 : xbsIndex_r4/Constant  const=1  gui_display_data_type=Fixed-point  arith_type=Unsigned  n_bits=1  bin_pt=0  preci_type=Single  exp_width=8  frac_width=24  explicit_period=off  period=1  equ=P=C  opselect=C  inp2=PCIN>>17  opr=+  inp1=P  carry=CIN  dbl_ovrd=off  block_type=constant
  Equal : Subsystem
  Mux : xbsIndex_r4/Mux  inputs=4  en=off  latency=0  precision=Full  arith_type=Unsigned  n_bits=16  bin_pt=14  quantization=Truncate  overflow=Wrap  dbl_ovrd=off  block_type=mux
  Mux1 : xbsIndex_r4/Mux  inputs=4  en=off  latency=0  precision=Full  arith_type=Unsigned  n_bits=16  bin_pt=14  quantization=Truncate  overflow=Wrap  dbl_ovrd=off  block_type=mux
  Not Equal : Subsystem
  Res : Outport
  Or Op : Outport  Port=2
  wires:
  Constant4/1 -> Mux1/5
  Constant3/1 -> Mux1/4
  Constant2/1 -> Mux1/3
  Constant1/1 -> Mux1/2
  Mux1/1 -> Or Op/1
  2LSB/1 -> Mux1/1, Mux/1
  Template/1 -> Any of AND/2(T), Not Equal/2(BT), Equal/2(BT)
  Data/1 -> Any of AND/1(D), Not Equal/1(D), Equal/1(D)
  Any of AND/1(R) -> Mux/5
  Not Equal/1(R) -> Mux/4
  Equal/1(R) -> Mux/3
  Constant/1 -> Mux/2
  Mux/1 -> Res/1
  Op/1 -> 2LSB/1

== system w3_warplab_trigger_proc/Trigger Sources/Ethernet/Pkt Comp/Word Comp 0/Subsystem ==
  32b : Inport
  8LSB+0 : xbsIndex_r4/Slice  nbits=8  boolean_output=off  mode=Lower Bit Location + Width  bit1=0  base1=MSB of Input  bit0=0  base0=LSB of Input  dbl_ovrd=off  block_type=slice
  8LSB+16 : xbsIndex_r4/Slice  nbits=8  boolean_output=off  mode=Lower Bit Location + Width  bit1=0  base1=MSB of Input  bit0=16  base0=LSB of Input  dbl_ovrd=off  block_type=slice
  8LSB+24 : xbsIndex_r4/Slice  nbits=8  boolean_output=off  mode=Lower Bit Location + Width  bit1=0  base1=MSB of Input  bit0=24  base0=LSB of Input  dbl_ovrd=off  block_type=slice
  8LSB+8 : xbsIndex_r4/Slice  nbits=8  boolean_output=off  mode=Lower Bit Location + Width  bit1=0  base1=MSB of Input  bit0=8  base0=LSB of Input  dbl_ovrd=off  block_type=slice
  B0 : Outport
  B1 : Outport  Port=2
  B2 : Outport  Port=3
  B3 : Outport  Port=4
  wires:
  32b/1 -> 8LSB+0/1, 8LSB+8/1, 8LSB+16/1, 8LSB+24/1
  8LSB+0/1 -> B0/1
  8LSB+8/1 -> B1/1
  8LSB+16/1 -> B2/1
  8LSB+24/1 -> B3/1

== system w3_warplab_trigger_proc/Trigger Sources/Ethernet/Pkt Comp/Word Comp 0/Subsystem1 ==
  32b : Inport
  8LSB+0 : xbsIndex_r4/Slice  nbits=8  boolean_output=off  mode=Lower Bit Location + Width  bit1=0  base1=MSB of Input  bit0=0  base0=LSB of Input  dbl_ovrd=off  block_type=slice
  8LSB+16 : xbsIndex_r4/Slice  nbits=8  boolean_output=off  mode=Lower Bit Location + Width  bit1=0  base1=MSB of Input  bit0=16  base0=LSB of Input  dbl_ovrd=off  block_type=slice
  8LSB+24 : xbsIndex_r4/Slice  nbits=8  boolean_output=off  mode=Lower Bit Location + Width  bit1=0  base1=MSB of Input  bit0=24  base0=LSB of Input  dbl_ovrd=off  block_type=slice
  8LSB+8 : xbsIndex_r4/Slice  nbits=8  boolean_output=off  mode=Lower Bit Location + Width  bit1=0  base1=MSB of Input  bit0=8  base0=LSB of Input  dbl_ovrd=off  block_type=slice
  B0 : Outport
  B1 : Outport  Port=2
  B2 : Outport  Port=3
  B3 : Outport  Port=4
  wires:
  8LSB+24/1 -> B3/1
  8LSB+16/1 -> B2/1
  8LSB+8/1 -> B1/1
  8LSB+0/1 -> B0/1
  32b/1 -> 8LSB+24/1, 8LSB+16/1, 8LSB+8/1, 8LSB+0/1

== system w3_warplab_trigger_proc/Trigger Sources/Ethernet/Pkt Comp/Word Comp 0/Subsystem2 ==
  32b : Inport
  8LSB+0 : xbsIndex_r4/Slice  nbits=8  boolean_output=off  mode=Lower Bit Location + Width  bit1=0  base1=MSB of Input  bit0=0  base0=LSB of Input  dbl_ovrd=off  block_type=slice
  8LSB+16 : xbsIndex_r4/Slice  nbits=8  boolean_output=off  mode=Lower Bit Location + Width  bit1=0  base1=MSB of Input  bit0=16  base0=LSB of Input  dbl_ovrd=off  block_type=slice
  8LSB+24 : xbsIndex_r4/Slice  nbits=8  boolean_output=off  mode=Lower Bit Location + Width  bit1=0  base1=MSB of Input  bit0=24  base0=LSB of Input  dbl_ovrd=off  block_type=slice
  8LSB+8 : xbsIndex_r4/Slice  nbits=8  boolean_output=off  mode=Lower Bit Location + Width  bit1=0  base1=MSB of Input  bit0=8  base0=LSB of Input  dbl_ovrd=off  block_type=slice
  B0 : Outport
  B1 : Outport  Port=2
  B2 : Outport  Port=3
  B3 : Outport  Port=4
  wires:
  32b/1 -> 8LSB+0/1, 8LSB+8/1, 8LSB+16/1, 8LSB+24/1
  8LSB+0/1 -> B0/1
  8LSB+8/1 -> B1/1
  8LSB+16/1 -> B2/1
  8LSB+24/1 -> B3/1

== system w3_warplab_trigger_proc/Trigger Sources/Energy/AntA Detector/Running Sum/Long Reset Gen/S-R Latch ==
  S : Inport
  R : Inport  Port=2
  Constant1 : xbsIndex_r4/Constant  const=1  gui_display_data_type=Fixed-point  arith_type=Boolean  n_bits=1  bin_pt=0  preci_type=Single  exp_width=8  frac_width=24  explicit_period=off  period=1  equ=P=C  opselect=C  inp2=PCIN>>17  opr=+  inp1=P  carry=CIN  dbl_ovrd=off  block_type=constant
      settings: block_version=VER_STRING_GOES_HERE
  Register2 : xbsIndex_r4/Register  init=0  rst=on  en=on  dbl_ovrd=off  block_type=register
      settings: xl_area=[1 1 0 0 0 0 0]  block_version=VER_STRING_GOES_HERE
  Q : Outport
  wires:
  Constant1/1 -> Register2/1
  R/1 -> Register2/2
  Register2/1 -> Q/1
  S/1 -> Register2/3

== system w3_warplab_trigger_proc/Trigger Sources/Energy/AntB Detector/Running Sum/Long Reset Gen/S-R Latch ==
  S : Inport
  R : Inport  Port=2
  Constant1 : xbsIndex_r4/Constant  const=1  gui_display_data_type=Fixed-point  arith_type=Boolean  n_bits=1  bin_pt=0  preci_type=Single  exp_width=8  frac_width=24  explicit_period=off  period=1  equ=P=C  opselect=C  inp2=PCIN>>17  opr=+  inp1=P  carry=CIN  dbl_ovrd=off  block_type=constant
      settings: block_version=VER_STRING_GOES_HERE
  Register2 : xbsIndex_r4/Register  init=0  rst=on  en=on  dbl_ovrd=off  block_type=register
      settings: xl_area=[1 1 0 0 0 0 0]  block_version=VER_STRING_GOES_HERE
  Q : Outport
  wires:
  S/1 -> Register2/3
  Register2/1 -> Q/1
  R/1 -> Register2/2
  Constant1/1 -> Register2/1

== system w3_warplab_trigger_proc/Trigger Sources/Energy/AntC Detector/Running Sum/Long Reset Gen/S-R Latch ==
  S : Inport
  R : Inport  Port=2
  Constant1 : xbsIndex_r4/Constant  const=1  gui_display_data_type=Fixed-point  arith_type=Boolean  n_bits=1  bin_pt=0  preci_type=Single  exp_width=8  frac_width=24  explicit_period=off  period=1  equ=P=C  opselect=C  inp2=PCIN>>17  opr=+  inp1=P  carry=CIN  dbl_ovrd=off  block_type=constant
      settings: block_version=VER_STRING_GOES_HERE
  Register2 : xbsIndex_r4/Register  init=0  rst=on  en=on  dbl_ovrd=off  block_type=register
      settings: xl_area=[1 1 0 0 0 0 0]  block_version=VER_STRING_GOES_HERE
  Q : Outport
  wires:
  Constant1/1 -> Register2/1
  R/1 -> Register2/2
  Register2/1 -> Q/1
  S/1 -> Register2/3

== system w3_warplab_trigger_proc/Trigger Sources/Energy/AntD Detector/Running Sum/Long Reset Gen/S-R Latch ==
  S : Inport
  R : Inport  Port=2
  Constant1 : xbsIndex_r4/Constant  const=1  gui_display_data_type=Fixed-point  arith_type=Boolean  n_bits=1  bin_pt=0  preci_type=Single  exp_width=8  frac_width=24  explicit_period=off  period=1  equ=P=C  opselect=C  inp2=PCIN>>17  opr=+  inp1=P  carry=CIN  dbl_ovrd=off  block_type=constant
      settings: block_version=VER_STRING_GOES_HERE
  Register2 : xbsIndex_r4/Register  init=0  rst=on  en=on  dbl_ovrd=off  block_type=register
      settings: xl_area=[1 1 0 0 0 0 0]  block_version=VER_STRING_GOES_HERE
  Q : Outport
  wires:
  S/1 -> Register2/3
  Register2/1 -> Q/1
  R/1 -> Register2/2
  Constant1/1 -> Register2/1

== system w3_warplab_trigger_proc/Trigger Sources/Ethernet/Pkt Comp/Word Comp 0/Byte Comp 0/Any of AND ==
  D : Inport
  T : Inport  Port=2
  Constant3 : xbsIndex_r4/Constant  const=0  gui_display_data_type=Fixed-point  arith_type=Unsigned  n_bits=8  bin_pt=0  preci_type=Single  exp_width=8  frac_width=24  explicit_period=off  period=1  equ=P=C  opselect=C  inp2=PCIN>>17  opr=+  inp1=P  carry=CIN  dbl_ovrd=off  block_type=constant
  Logical : xbsIndex_r4/Logical  logical_function=AND  inputs=2  en=off  latency=0  precision=Full  arith_type=Unsigned  n_bits=16  bin_pt=0  align_bp=on  dbl_ovrd=off  block_type=logical
  Relational1 : xbsIndex_r4/Relational  mode=a!=b  en=off  latency=0  dbl_ovrd=off  block_type=relational
  R : Outport
  wires:
  Constant3/1 -> Relational1/1
  Logical/1 -> Relational1/2
  D/1 -> Logical/1
  T/1 -> Logical/2
  Relational1/1 -> R/1

== system w3_warplab_trigger_proc/Trigger Sources/Ethernet/Pkt Comp/Word Comp 0/Byte Comp 0/Equal ==
  D : Inport
  BT : Inport  Port=2
  Relational : xbsIndex_r4/Relational  mode=a=b  en=off  latency=0  dbl_ovrd=off  block_type=relational
  R : Outport
  wires:
  D/1 -> Relational/1
  BT/1 -> Relational/2
  Relational/1 -> R/1

== system w3_warplab_trigger_proc/Trigger Sources/Ethernet/Pkt Comp/Word Comp 0/Byte Comp 0/Not Equal ==
  D : Inport
  BT : Inport  Port=2
  Relational : xbsIndex_r4/Relational  mode=a!=b  en=off  latency=0  dbl_ovrd=off  block_type=relational
  R : Outport
  wires:
  Relational/1 -> R/1
  BT/1 -> Relational/2
  D/1 -> Relational/1

== system w3_warplab_trigger_proc/Trigger Sources/Ethernet/Pkt Comp/Word Comp 0/Byte Comp 1/Any of AND ==
  D : Inport
  T : Inport  Port=2
  Constant3 : xbsIndex_r4/Constant  const=0  gui_display_data_type=Fixed-point  arith_type=Unsigned  n_bits=8  bin_pt=0  preci_type=Single  exp_width=8  frac_width=24  explicit_period=off  period=1  equ=P=C  opselect=C  inp2=PCIN>>17  opr=+  inp1=P  carry=CIN  dbl_ovrd=off  block_type=constant
  Logical : xbsIndex_r4/Logical  logical_function=AND  inputs=2  en=off  latency=0  precision=Full  arith_type=Unsigned  n_bits=16  bin_pt=0  align_bp=on  dbl_ovrd=off  block_type=logical
  Relational1 : xbsIndex_r4/Relational  mode=a!=b  en=off  latency=0  dbl_ovrd=off  block_type=relational
  R : Outport
  wires:
  Relational1/1 -> R/1
  T/1 -> Logical/2
  D/1 -> Logical/1
  Logical/1 -> Relational1/2
  Constant3/1 -> Relational1/1

== system w3_warplab_trigger_proc/Trigger Sources/Ethernet/Pkt Comp/Word Comp 0/Byte Comp 1/Equal ==
  D : Inport
  BT : Inport  Port=2
  Relational : xbsIndex_r4/Relational  mode=a=b  en=off  latency=0  dbl_ovrd=off  block_type=relational
  R : Outport
  wires:
  Relational/1 -> R/1
  BT/1 -> Relational/2
  D/1 -> Relational/1

== system w3_warplab_trigger_proc/Trigger Sources/Ethernet/Pkt Comp/Word Comp 0/Byte Comp 1/Not Equal ==
  D : Inport
  BT : Inport  Port=2
  Relational : xbsIndex_r4/Relational  mode=a!=b  en=off  latency=0  dbl_ovrd=off  block_type=relational
  R : Outport
  wires:
  D/1 -> Relational/1
  BT/1 -> Relational/2
  Relational/1 -> R/1

== system w3_warplab_trigger_proc/Trigger Sources/Ethernet/Pkt Comp/Word Comp 0/Byte Comp 2/Any of AND ==
  D : Inport
  T : Inport  Port=2
  Constant3 : xbsIndex_r4/Constant  const=0  gui_display_data_type=Fixed-point  arith_type=Unsigned  n_bits=8  bin_pt=0  preci_type=Single  exp_width=8  frac_width=24  explicit_period=off  period=1  equ=P=C  opselect=C  inp2=PCIN>>17  opr=+  inp1=P  carry=CIN  dbl_ovrd=off  block_type=constant
  Logical : xbsIndex_r4/Logical  logical_function=AND  inputs=2  en=off  latency=0  precision=Full  arith_type=Unsigned  n_bits=16  bin_pt=0  align_bp=on  dbl_ovrd=off  block_type=logical
  Relational1 : xbsIndex_r4/Relational  mode=a!=b  en=off  latency=0  dbl_ovrd=off  block_type=relational
  R : Outport
  wires:
  Constant3/1 -> Relational1/1
  Logical/1 -> Relational1/2
  D/1 -> Logical/1
  T/1 -> Logical/2
  Relational1/1 -> R/1

== system w3_warplab_trigger_proc/Trigger Sources/Ethernet/Pkt Comp/Word Comp 0/Byte Comp 2/Equal ==
  D : Inport
  BT : Inport  Port=2
  Relational : xbsIndex_r4/Relational  mode=a=b  en=off  latency=0  dbl_ovrd=off  block_type=relational
  R : Outport
  wires:
  D/1 -> Relational/1
  BT/1 -> Relational/2
  Relational/1 -> R/1

== system w3_warplab_trigger_proc/Trigger Sources/Ethernet/Pkt Comp/Word Comp 0/Byte Comp 2/Not Equal ==
  D : Inport
  BT : Inport  Port=2
  Relational : xbsIndex_r4/Relational  mode=a!=b  en=off  latency=0  dbl_ovrd=off  block_type=relational
  R : Outport
  wires:
  Relational/1 -> R/1
  BT/1 -> Relational/2
  D/1 -> Relational/1

== system w3_warplab_trigger_proc/Trigger Sources/Ethernet/Pkt Comp/Word Comp 0/Byte Comp 3/Any of AND ==
  D : Inport
  T : Inport  Port=2
  Constant3 : xbsIndex_r4/Constant  const=0  gui_display_data_type=Fixed-point  arith_type=Unsigned  n_bits=8  bin_pt=0  preci_type=Single  exp_width=8  frac_width=24  explicit_period=off  period=1  equ=P=C  opselect=C  inp2=PCIN>>17  opr=+  inp1=P  carry=CIN  dbl_ovrd=off  block_type=constant
  Logical : xbsIndex_r4/Logical  logical_function=AND  inputs=2  en=off  latency=0  precision=Full  arith_type=Unsigned  n_bits=16  bin_pt=0  align_bp=on  dbl_ovrd=off  block_type=logical
  Relational1 : xbsIndex_r4/Relational  mode=a!=b  en=off  latency=0  dbl_ovrd=off  block_type=relational
  R : Outport
  wires:
  Relational1/1 -> R/1
  T/1 -> Logical/2
  D/1 -> Logical/1
  Logical/1 -> Relational1/2
  Constant3/1 -> Relational1/1

== system w3_warplab_trigger_proc/Trigger Sources/Ethernet/Pkt Comp/Word Comp 0/Byte Comp 3/Equal ==
  D : Inport
  BT : Inport  Port=2
  Relational : xbsIndex_r4/Relational  mode=a=b  en=off  latency=0  dbl_ovrd=off  block_type=relational
  R : Outport
  wires:
  Relational/1 -> R/1
  BT/1 -> Relational/2
  D/1 -> Relational/1

== system w3_warplab_trigger_proc/Trigger Sources/Ethernet/Pkt Comp/Word Comp 0/Byte Comp 3/Not Equal ==
  D : Inport
  BT : Inport  Port=2
  Relational : xbsIndex_r4/Relational  mode=a!=b  en=off  latency=0  dbl_ovrd=off  block_type=relational
  R : Outport
  wires:
  D/1 -> Relational/1
  BT/1 -> Relational/2
  Relational/1 -> R/1
